simulink model "car_statemachine"  (Simulink 6.4)
settings: Solver=ode45  StartTime=0.0  StopTime=30.0  RelTol=1e-3
model workspace (MAT data in the model file):
  Vup = [10  30  50  1000000; 10  30  50  1000000; 15  30  50  1000000; 23  41  60  1000000; 40  70  100  1000000; 40  70  100  1000000]
  Vdown = [0  5  20  35; 0  5  20  35; 0  5  25  40; 0  5  30  50; 0  30  50  80; 0  30  50  80]
  THup = [0; 25; 35; 50; 90; 100]
  THdown = [0; 5; 40; 50; 90; 100]
  TH = [0; 20; 30; 40; 50; 60; 70; 80; 90; 100]
  Te = [-40  -44  -49  -53  -57  -61  -65  -70  -74  -78  -82; 215  117  85  66  44  29  10  -2  -13  -22  -32; 245  208  178  148  122  104  85  66  48  33  18; 264  260  241  219  193  167  152  133  119  96  85; 264  279  282  275  260  238  223  208  189  171  152; 267  290  293  297  290  275  260  256  234  212  193; 267  297  305  305  305  301  293  282  267  249  226; 267  301  308  312  319  323  319  316  297  279  253; 267  301  312  319  327  327  327  327  312  293  267; 267  301  312  319  327  334  334  334  319  305  275]
  Rw = 1
  Qt = [2.232; 2.075; 1.975; 1.846; 1.72; 1.564; 1.409; 1.254; 1.096; 1.08; 1.061; 1.043; 1.028; 1.012; 1.002; 1.002; 1.001; 0.998; 0.999; 1.001; 1.002]
  Qn = [0; 0.1; 0.2; 0.3; 0.4; 0.5; 0.6; 0.7; 0.8; 0.81; 0.82; 0.83; 0.84; 0.85; 0.86; 0.87; 0.88; 0.89; 0.9; 0.92; 0.94]
  Qfd = 3.23
  Ne = [800 1200 1600 2000 2400 2800 3200 3600 4000 4400 4800]
  K = [137.465208994; 137.065019157; 135.864449646; 135.664354728; 137.565256453; 140.366585312; 145.268910814; 152.872517717; 162.9773111; 164.27792807; 166.178829795; 167.979684062; 170.080680706; 172.781962105; 175.383196045; 179.585189333; 183.587087703; 189.890077635; 197.693779455; 215.902417037; 244.515990379]
  Iv = 12.0941478573
  Ie = 0.0219914882836
  F = 40
  Cd : num (value not decoded)
undefined symbols (not defined in the file or in its folder): sigbuilder_block
settings Model: Creator=oqaqish  LastModifiedBy=rsnah
settings DataIOCC: SignalLoggingName=sigsOut
settings OptimizationCC: InlineInvariantSignals=on
settings DebuggingCC: CheckExecutionContextPreStartOutputMsg=on  CheckExecutionContextRuntimeOutputMsg=on  SolverPrmCheckMsg=none  StrictBusMsg=None
settings HardwareCC: TargetUnknown=on
settings GRTTargetCC: ModelReferenceCompliant=off  MatFileLogging=off

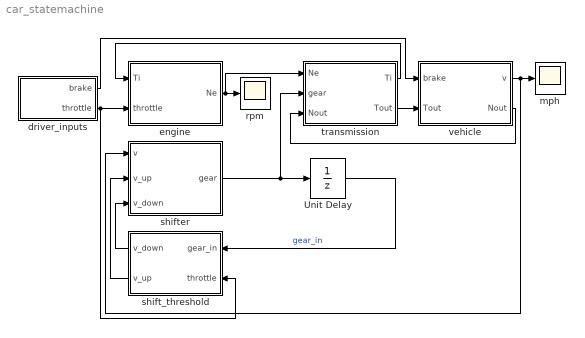
== system car_statemachine ==
  Unit Delay : UnitDelay  X0=1  SampleTime=0.05
      settings: AttributesFormatString=Ts = %<SampleTime>\n
  driver_inputs : Subsystem  Tag=STV Subsys  LoadFcn=sigbuilder_block('load');  StartFcn=sigbuilder_block('start');  StopFcn=sigbuilder_block('stop');  ClipboardFcn=sigbuilder_block('clipboard');  mask(Sigbuilder block){}
      mask help: Sigbuilder GUI
      mask init:
      | tuvar = sigbuilder_block('maskInit');
      settings: CopyFcn=sigbuilder_block('copy');  DeleteFcn=sigbuilder_block('delete');  ModelCloseFcn=sigbuilder_block('modelClose');  PreSaveFcn=sigbuilder_block('preSave');  NameChangeFcn=sigbuilder_block('namechange');  OpenFcn=sigbuilder_block('open',[113.25 99.75 519.75 399.75 ]);  CloseFcn=sigbuilder_block('close');
      mask Display: plot(0,0,100,100,[10,10,40,40,10],[80,20,20,80,80],[40,10],[50,50], [40,27,10],[65,72,56],[40,25,25,10],[28,28,43,43]);
  engine : Subsystem
  mph : Scope
      settings: TimeRange=30  YMin=0  YMax=140
  rpm : Scope
      settings: TimeRange=30  YMin=1000  YMax=6000
  shift_threshold : Subsystem  Orientation=left
  shifter : Stateflow chart
  transmission : Subsystem
  vehicle : Subsystem
  wires:
  driver_inputs/2(throttle) -> shift_threshold/2(throttle), engine/2(throttle)
  engine/1(Ne) -> transmission/1(Ne), rpm/1
  transmission/1(Ti) -> engine/1(Ti)
  driver_inputs/1(brake) -> vehicle/1(brake)
  transmission/2(Tout) -> vehicle/2(Tout)
  Unit Delay/1 -> shift_threshold/1(gear_in)  "gear_in"
  shift_threshold/1(v_down) -> shifter/3(v_down)
  shift_threshold/2(v_up) -> shifter/2(v_up)
  vehicle/2(Nout) -> transmission/3(Nout)
  vehicle/1(v) -> mph/1, shifter/1(v)
  shifter/1(gear) -> Unit Delay/1, transmission/2(gear)

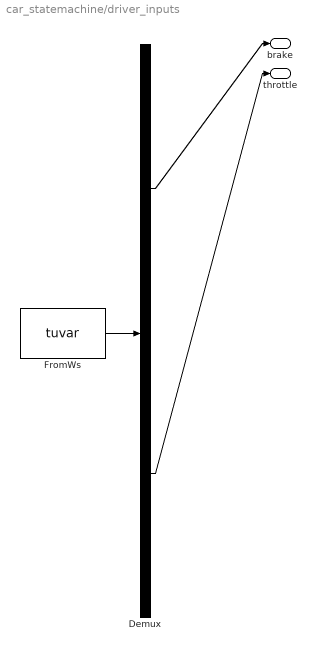
== system car_statemachine/driver_inputs ==
  Demux : Demux  Tag=STV Demux  Outputs=2
  FromWs : FromWorkspace  Tag=STV FromWs  VariableName=tuvar  SampleTime=0  SigBuilderData=DataTag1  VnvData=DataTag2
      SigBuilderData=|
      | channels(1).label = 'brake'
      | channels(1).allXData = {[0 50]}
      | channels(1).allYData = {[0 0]}
      | channels(2).label = 'throttle'
      | channels(2).allXData = {[0 15 15 50]}
      | channels(2).allYData = {[60 40 100 60]}
      | dataSet.timeRange = [0 50]
      | dataSet.name = 'Passing Manuver'
  brake : Outport  Tag=STV Outport
  throttle : Outport  Tag=STV Outport  Port=2
  wires:
  Demux/2 -> throttle/1
  Demux/1 -> brake/1
  FromWs/1 -> Demux/1

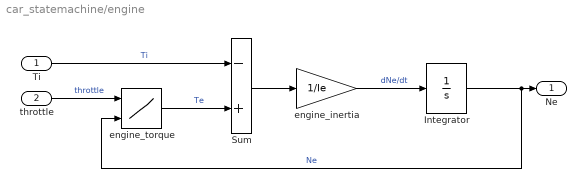
== system car_statemachine/engine ==
  Ti : Inport
  throttle : Inport  Port=2
  Integrator : Integrator  InitialCondition=1000  LimitOutput=on  UpperSaturationLimit=6000  LowerSaturationLimit=600  ZeroCross=off
      settings: AttributesFormatString="Ne0 = %<InitialCondition>\\n%<LowerSaturationLimit> <= Ne <=  %<UpperSaturationLimit>\\n\\n"
  Sum : Sum  Inputs=-+  SaturateOnIntegerOverflow=on  InputSameDT=on
  engine_inertia : Gain  Gain=1/Ie  SaturateOnIntegerOverflow=on
  engine_torque : Lookup2D  RowIndex=TH  ColumnIndex=Ne  OutputValues=Te  SaturateOnIntegerOverflow=on
  Ne : Outport
  wires:
  Sum/1 -> engine_inertia/1
  throttle/1 -> engine_torque/1  "throttle"
  engine_torque/1 -> Sum/2  "Te"
  Ti/1 -> Sum/1  "Ti"
  Integrator/1 -> Ne/1, engine_torque/2  "Ne"
  engine_inertia/1 -> Integrator/1  "dNe/dt"

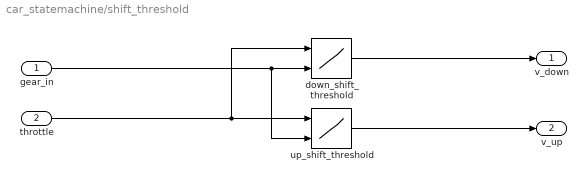
== system car_statemachine/shift_threshold ==
  gear_in : Inport
  throttle : Inport  Port=2
  down_shift_threshold : Lookup2D  RowIndex=THdown  ColumnIndex=[1:4]  OutputValues=Vdown  OutScaling=2^-10  InputSameDT=on
  up_shift_threshold : Lookup2D  RowIndex=THup  ColumnIndex=[1:4]  OutputValues=Vup  OutScaling=2^-10  InputSameDT=on
  v_down : Outport
  v_up : Outport  Port=2
  wires:
  up_shift_threshold/1 -> v_up/1
  down_shift_threshold/1 -> v_down/1
  throttle/1 -> up_shift_threshold/1, down_shift_threshold/1
  gear_in/1 -> up_shift_threshold/2, down_shift_threshold/2

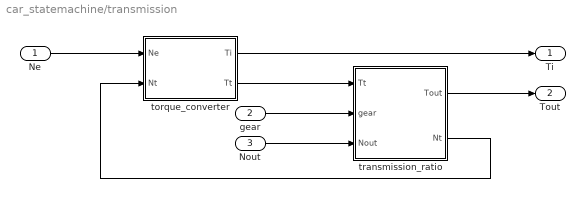
== system car_statemachine/transmission ==
  Ne : Inport
  gear : Inport  Port=2
  Nout : Inport  Port=3
  torque_converter : Subsystem
  transmission_ratio : Subsystem
  Ti : Outport  InitialOutput=0
  Tout : Outport  Port=2  InitialOutput=0
  wires:
  transmission_ratio/2(Nt) -> torque_converter/2(Nt)
  Ne/1 -> torque_converter/1(Ne)
  gear/1 -> transmission_ratio/2(gear)
  Nout/1 -> transmission_ratio/3(Nout)
  transmission_ratio/1(Tout) -> Tout/1
  torque_converter/2(Tt) -> transmission_ratio/1(Tt)
  torque_converter/1(Ti) -> Ti/1

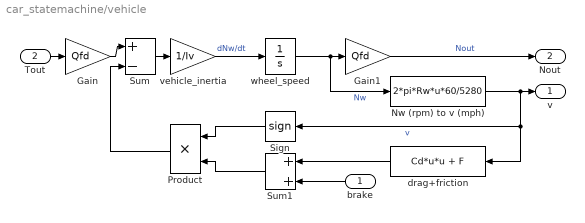
== system car_statemachine/vehicle ==
  brake : Inport  Orientation=left
  Tout : Inport  Port=2
  Gain : Gain  Gain=Qfd  SaturateOnIntegerOverflow=on
  Gain1 : Gain  Gain=Qfd  SaturateOnIntegerOverflow=on
  Nw (rpm) to v (mph) : Fcn  Expr=2*pi*Rw*u*60/5280
  Product : Product  Orientation=left  SaturateOnIntegerOverflow=on
  Sign : Signum  Orientation=left
  Sum : Sum  Inputs=|+-  SaturateOnIntegerOverflow=on
  Sum1 : Sum  Orientation=left  SaturateOnIntegerOverflow=on
  drag+friction : Fcn  Orientation=left  Expr=Cd*u*u + F
  vehicle_inertia : Gain  Gain=1/Iv  SaturateOnIntegerOverflow=on
  wheel_speed : Integrator
      settings: AttributesFormatString=Nw0 = %<InitialCondition>\n
  v : Outport
  Nout : Outport  Port=2
  wires:
  Tout/1 -> Gain/1
  Gain/1 -> Sum/1
  Sum/1 -> vehicle_inertia/1
  wheel_speed/1 -> Gain1/1, Nw (rpm) to v (mph)/1  "Nw"
  Gain1/1 -> Nout/1  "Nout"
  Nw (rpm) to v (mph)/1 -> v/1, Sign/1, drag+friction/1  "v"
  vehicle_inertia/1 -> wheel_speed/1  "dNw/dt"
  brake/1 -> Sum1/2
  drag+friction/1 -> Sum1/1
  Sign/1 -> Product/1
  Sum1/1 -> Product/2
  Product/1 -> Sum/2

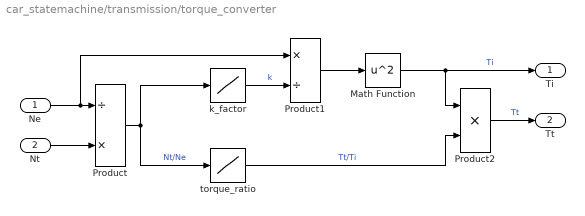
== system car_statemachine/transmission/torque_converter ==
  Ne : Inport
  Nt : Inport  Port=2
  Math Function : Math  Operator=square  SaturateOnIntegerOverflow=on
  Product : Product  Inputs=/*  SaturateOnIntegerOverflow=on
  Product1 : Product  Inputs=*/  SaturateOnIntegerOverflow=on
  Product2 : Product  Inputs=**  SaturateOnIntegerOverflow=on
  k_factor : Lookup  InputValues=Qn  OutputValues=K  SaturateOnIntegerOverflow=on
  torque_ratio : Lookup  InputValues=Qn  OutputValues=Qt  SaturateOnIntegerOverflow=on
  Ti : Outport
  Tt : Outport  Port=2
  wires:
  Product1/1 -> Math Function/1
  torque_ratio/1 -> Product2/2  "Tt/Ti"
  Math Function/1 -> Product2/1, Ti/1  "Ti"
  k_factor/1 -> Product1/2  "k"
  Product/1 -> k_factor/1, torque_ratio/1  "Nt/Ne"
  Ne/1 -> Product1/1, Product/1
  Product2/1 -> Tt/1  "Tt"
  Nt/1 -> Product/2

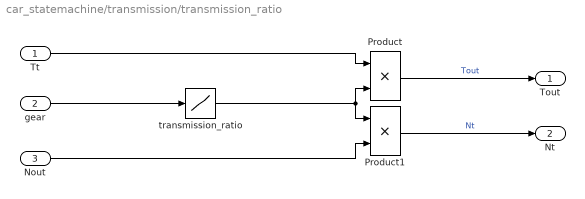
== system car_statemachine/transmission/transmission_ratio ==
  Tt : Inport
  gear : Inport  Port=2
  Nout : Inport  Port=3
  Product : Product  SaturateOnIntegerOverflow=on  InputSameDT=on
  Product1 : Product  SaturateOnIntegerOverflow=on  InputSameDT=on
  transmission_ratio : Lookup  InputValues=[1, 2, 3, 4]  OutputValues=[2.393, 1.450, 1.000, 0.677]  SaturateOnIntegerOverflow=on
  Tout : Outport  InitialOutput=0
  Nt : Outport  Port=2  InitialOutput=0
  wires:
  gear/1 -> transmission_ratio/1
  Tt/1 -> Product/1
  Product/1 -> Tout/1  "Tout"
  Product1/1 -> Nt/1  "Nt"
  Nout/1 -> Product1/2
  transmission_ratio/1 -> Product1/1, Product/2

== stateflow chart shifter ==
  settings: updateMethod=DISCRETE  sampleTime=0.05
  state Gear_1
    en: gear = 1;
  state Gear_2
    en: gear = 2;
  state Gear_3
    en: gear = 3;
  state Gear_4
    en: gear = 4;
  Gear_2 -> Gear_1 [order 2] : [v < v_down]
  Gear_1 -> Gear_2 : [v > v_up]
  Gear_2 -> Gear_3 [order 1] : [v > v_up]
  Gear_3 -> Gear_4 [order 1] : [v > v_up]
  Gear_4 -> Gear_3 : [v < v_down]
  Gear_3 -> Gear_2 [order 2] : [v < v_down]
  (default) -> Gear_1
  data: v input double; v_up input double; v_down input double; gear output double =1
